simulink model "gtm_aeromodel"  (Simulink 7.2)
settings: Solver=ode45  StartTime=0.0  StopTime=10.0  RelTol=1e-3
undefined symbols (not defined in the file or in its folder): A_BLCG, A_BW, A_CW, A_FSCG, A_FSREF_in, A_SW, A_WLCG, A_WLREF, ALPHA0, bclowb, bclowbx_FMACH, bcmowb, bcmowbx_FHP, bcmowby_FMACH, cda, cdax_FLPDEF, cddr, cddrx_FMACH, cdo, cdox_FLPDEF, cdt1, cdt1x_mach, cdt2, cdt2x_mach, cdto, cdtox_mach, cdwb, cdwbx_FALPHA, cdwby_FMACH, clat, clatfr, clatfrx_FHP, clatfry_FMACH, clatx_mach, clawbfr, clawbfrx_FHP, clawbfry_FMACH, cldefr, cldefrx_FHP, cldefry_FMACH, cldtab, cldtabx_FMACH, clqwb, clqwbfr, clqwbfrx_FHP, clqwbfry_FMACH, clqwbx_mach, cltdd, cltddx_FHP, cltddy_FMACH, clwb, clwbtdd, clwbtddx_FHP, clwbtddy_FMACH, clwbx_FALPHA, clwby_FMACH, clwbzdd, clwbzddx_FHP, clwbzddy_FMACH, clzdd ... (+196)
libraries: model_lib x1
(part 5 of 10)

== system gtm_aeromodel/get aero forces and moments/AERODYNAMICS/Force  Coefficients/SIDE/CYSPOIL ==
  dsb : Inport  OutDataType=sfix(16)  OutScaling=2^0
  dsl : Inport  Port=2  OutDataType=sfix(16)  OutScaling=2^0
  alpha : Inport  Port=3  OutDataType=sfix(16)  OutScaling=2^0
  mach : Inport  Port=4  OutDataType=sfix(16)  OutScaling=2^0
  flap : Inport  Port=5  OutDataType=sfix(16)  OutScaling=2^0
  dsr : Inport  Port=6  OutDataType=sfix(16)  OutScaling=2^0
  MACH : Constant  Value=.178  OutDataType=sfix(16)  OutScaling=2^0
  Sum1 : Sum  Inputs=-+  OutDataType=sfix(16)  OutScaling=2^0  SaturateOnIntegerOverflow=on  InputSameDT=on  OutDataTypeStr=Inherit: Same as first input
  Sum2 : Sum  OutDataType=sfix(16)  OutScaling=2^0  SaturateOnIntegerOverflow=on  InputSameDT=on  OutDataTypeStr=Inherit: Same as first input
  Sum5 : Sum  Inputs=+-  OutDataType=sfix(16)  OutScaling=2^0  SaturateOnIntegerOverflow=on  InputSameDT=on  OutDataTypeStr=Inherit: Same as first input
  Sum6 : Sum  Inputs=+-  OutDataType=sfix(16)  OutScaling=2^0  SaturateOnIntegerOverflow=on  InputSameDT=on  OutDataTypeStr=Inherit: Same as first input
  Sum7 : Sum  Inputs=+-  OutDataType=sfix(16)  OutScaling=2^0  SaturateOnIntegerOverflow=on  InputSameDT=on  OutDataTypeStr=Inherit: Same as first input
  Switch7 : Switch  Threshold=0.5  SaturateOnIntegerOverflow=on  InputSameDT=on
  cy_sp_int : Subsystem  TreatAsAtomicUnit=on
  dclpfint1 : Sum  Inputs=-+  OutDataType=sfix(16)  OutScaling=2^0  SaturateOnIntegerOverflow=on  InputSameDT=on  OutDataTypeStr=Inherit: Same as first input
  dclpfint2 : Sum  Inputs=-+  OutDataType=sfix(16)  OutScaling=2^0  SaturateOnIntegerOverflow=on  InputSameDT=on  OutDataTypeStr=Inherit: Same as first input
  dcyspfint : Sum  Inputs=-+  OutDataType=sfix(16)  OutScaling=2^0  SaturateOnIntegerOverflow=on  InputSameDT=on  OutDataTypeStr=Inherit: Same as first input
  dcywbdsl : Subsystem  mask(1-2-3 Table){@1=dcywbdsl_Fx_DSL, @2=dcywbdsl_Fy_FALPHA, @3=dcywbdsl_Fz_FMACH, @4=dcywbdsl_F}
      mask prompts: @1 "X vector:"; @2 "Y vector:"; @3 "Z vector:"; @4 "Table:"
      mask help: 3-D Table Look Up. Enter monotonic X, Y and Z vectors and a matrix of 2-D tables. See the help for more info.
      mask init:
      | x=@1;y=@2;z=@3;tab=@4;
      mask Help: The X, Y and Z vectors must be monotonic.   The 3-D table is a horizontal concatenation of  2-D tables.  X  indexes into the columns of the 2-D tables & Y indexes into the rows of the 2-D tables.  Z indexes into the table levels (starting with the 1st 2-D table).   The input values are x, y and z respectively (e.g., top port = x).
      mask Display: plot([0 2 2 0 0],[0 0 2 2 0],[0 2 2.9 0.95 0],[2 2 2.7 2.7 2],[2 2.9 2.9 2 2],[0 0.85 2.7 2 0])
  dcywbdsl1 : Subsystem  mask(1-2-3 Table){@1=dcywbdsl_Fx_DSL, @2=dcywbdsl_Fy_FALPHA, @3=dcywbdsl_Fz_FMACH, @4=dcywbdsl_F}
      mask prompts: @1 "X vector:"; @2 "Y vector:"; @3 "Z vector:"; @4 "Table:"
      mask help: 3-D Table Look Up. Enter monotonic X, Y and Z vectors and a matrix of 2-D tables. See the help for more info.
      mask init:
      | x=@1;y=@2;z=@3;tab=@4;
      mask Help: The X, Y and Z vectors must be monotonic.   The 3-D table is a horizontal concatenation of  2-D tables.  X  indexes into the columns of the 2-D tables & Y indexes into the rows of the 2-D tables.  Z indexes into the table levels (starting with the 1st 2-D table).   The input values are x, y and z respectively (e.g., top port = x).
      mask Display: plot([0 2 2 0 0],[0 0 2 2 0],[0 2 2.9 0.95 0],[2 2 2.7 2.7 2],[2 2.9 2.9 2 2],[0 0.85 2.7 2 0])
  dcywbdsl2 : Subsystem  mask(1-2-3 Table){@1=dcywbdsl_Fx_DSL, @2=dcywbdsl_Fy_FALPHA, @3=dcywbdsl_Fz_FMACH, @4=dcywbdsl_F}
      mask prompts: @1 "X vector:"; @2 "Y vector:"; @3 "Z vector:"; @4 "Table:"
      mask help: 3-D Table Look Up. Enter monotonic X, Y and Z vectors and a matrix of 2-D tables. See the help for more info.
      mask init:
      | x=@1;y=@2;z=@3;tab=@4;
      mask Help: The X, Y and Z vectors must be monotonic.   The 3-D table is a horizontal concatenation of  2-D tables.  X  indexes into the columns of the 2-D tables & Y indexes into the rows of the 2-D tables.  Z indexes into the table levels (starting with the 1st 2-D table).   The input values are x, y and z respectively (e.g., top port = x).
      mask Display: plot([0 2 2 0 0],[0 0 2 2 0],[0 2 2.9 0.95 0],[2 2 2.7 2.7 2],[2 2.9 2.9 2 2],[0 0.85 2.7 2 0])
  dcywbdsl3 : Subsystem  mask(1-2-3 Table){@1=dcywbdsl_Fx_DSL, @2=dcywbdsl_Fy_FALPHA, @3=dcywbdsl_Fz_FMACH, @4=dcywbdsl_F}
      mask prompts: @1 "X vector:"; @2 "Y vector:"; @3 "Z vector:"; @4 "Table:"
      mask help: 3-D Table Look Up. Enter monotonic X, Y and Z vectors and a matrix of 2-D tables. See the help for more info.
      mask init:
      | x=@1;y=@2;z=@3;tab=@4;
      mask Help: The X, Y and Z vectors must be monotonic.   The 3-D table is a horizontal concatenation of  2-D tables.  X  indexes into the columns of the 2-D tables & Y indexes into the rows of the 2-D tables.  Z indexes into the table levels (starting with the 1st 2-D table).   The input values are x, y and z respectively (e.g., top port = x).
      mask Display: plot([0 2 2 0 0],[0 0 2 2 0],[0 2 2.9 0.95 0],[2 2 2.7 2.7 2],[2 2.9 2.9 2 2],[0 0.85 2.7 2 0])
  dcywbdsl4 : Subsystem  mask(1-2-3 Table){@1=dcywbdsl_Fx_DSL, @2=dcywbdsl_Fy_FALPHA, @3=dcywbdsl_Fz_FMACH, @4=dcywbdsl_F}
      mask prompts: @1 "X vector:"; @2 "Y vector:"; @3 "Z vector:"; @4 "Table:"
      mask help: 3-D Table Look Up. Enter monotonic X, Y and Z vectors and a matrix of 2-D tables. See the help for more info.
      mask init:
      | x=@1;y=@2;z=@3;tab=@4;
      mask Help: The X, Y and Z vectors must be monotonic.   The 3-D table is a horizontal concatenation of  2-D tables.  X  indexes into the columns of the 2-D tables & Y indexes into the rows of the 2-D tables.  Z indexes into the table levels (starting with the 1st 2-D table).   The input values are x, y and z respectively (e.g., top port = x).
      mask Display: plot([0 2 2 0 0],[0 0 2 2 0],[0 2 2.9 0.95 0],[2 2 2.7 2.7 2],[2 2.9 2.9 2 2],[0 0.85 2.7 2 0])
  dcywbdsl5 : Subsystem  mask(1-2-3 Table){@1=dcywbdsl_Fx_DSL, @2=dcywbdsl_Fy_FALPHA, @3=dcywbdsl_Fz_FMACH, @4=dcywbdsl_F}
      mask prompts: @1 "X vector:"; @2 "Y vector:"; @3 "Z vector:"; @4 "Table:"
      mask help: 3-D Table Look Up. Enter monotonic X, Y and Z vectors and a matrix of 2-D tables. See the help for more info.
      mask init:
      | x=@1;y=@2;z=@3;tab=@4;
      mask Help: The X, Y and Z vectors must be monotonic.   The 3-D table is a horizontal concatenation of  2-D tables.  X  indexes into the columns of the 2-D tables & Y indexes into the rows of the 2-D tables.  Z indexes into the table levels (starting with the 1st 2-D table).   The input values are x, y and z respectively (e.g., top port = x).
      mask Display: plot([0 2 2 0 0],[0 0 2 2 0],[0 2 2.9 0.95 0],[2 2 2.7 2.7 2],[2 2.9 2.9 2 2],[0 0.85 2.7 2 0])
  zero : Constant  Value=0.0  OutDataType=sfix(16)  OutScaling=2^0
  cy_spoil : Outport  OutDataType=sfix(16)  OutScaling=2^0  InitialOutput=0
  wires:
  Sum6/1 -> Sum2/1
  dsb/1 -> dcywbdsl1/1(X), cy_sp_int/4(dsb), dcywbdsl3/1(X)
  zero/1 -> Switch7/3
  dcywbdsl2/1(Interp Value) -> Sum5/1
  Sum1/1 -> Sum6/1
  Sum5/1 -> Sum6/2
  dsl/1 -> dcywbdsl/1(X), cy_sp_int/3(dsl), dcywbdsl4/1(X)
  alpha/1 -> dcywbdsl/2(Y), dcywbdsl2/2(Y), dcywbdsl3/2(Y), cy_sp_int/2(alpha), dcywbdsl5/2(Y), dcywbdsl4/2(Y), dcywbdsl1/2(Y)
  dcywbdsl/1(Interp Value) -> Sum1/2
  mach/1 -> dcywbdsl/3(Z), dcywbdsl1/3(Z), dcywbdsl2/3(Z)
  dsr/1 -> dcywbdsl2/1(X), dcywbdsl5/1(X), cy_sp_int/5(dsr)
  dcywbdsl5/1(Interp Value) -> dclpfint1/2
  dcywbdsl3/1(Interp Value) -> dclpfint1/1, dclpfint2/1
  dcywbdsl4/1(Interp Value) -> dclpfint2/2
  dclpfint2/1 -> Sum7/1
  dclpfint1/1 -> Sum7/2
  Sum7/1 -> dcyspfint/1
  MACH/1 -> dcywbdsl5/3(Z), dcywbdsl4/3(Z), dcywbdsl3/3(Z)
  dcywbdsl1/1(Interp Value) -> Sum1/1, Sum5/2
  flap/1 -> cy_sp_int/Enable, Switch7/2, cy_sp_int/1(flap)
  cy_sp_int/1(cy_spfl_int) -> dcyspfint/2
  dcyspfint/1 -> Switch7/1
  Sum2/1 -> cy_spoil/1
  Switch7/1 -> Sum2/2

== system gtm_aeromodel/get aero forces and moments/AERODYNAMICS/Force  Coefficients/SIDE/TAIL ==
  mach : Inport  OutDataType=sfix(16)  OutScaling=2^0
  alpha : Inport  Port=2  OutDataType=sfix(16)  OutScaling=2^0
  Sum : Sum  OutDataType=sfix(16)  OutScaling=2^0  SaturateOnIntegerOverflow=on  InputSameDT=on  OutDataTypeStr=Inherit: Same as first input
  cybht : Subsystem  mask(2-D Table){y=cybhtx_FMACH, z=cybhty_FALPHA, tab=cybht}
      mask prompts: y "Y vector:"; z "Z vector:"; tab "Table:"
      mask help: 2-D Table Look Up. Enter monotonic Y and Z vectors and a matrix of 2-D tables. See the help for more info.
      mask Help: The Y and Z vectors must be monotonic.  Y  indexes into the columns of the 2-D table & Z indexes into the rows of the 2-D tables.   The input values are y and z respectively (e.g., top port = y).
      mask Display: plot(-10,-10,110,110,[90,50,10],[90,40,30],[90,50,10],[50,26,20],[90,50,10],[22,13,10])
  cybvt : Subsystem  mask(2-D Table){y=cybvtx_FMACH, z=cybvty_FALPHA, tab=cybvt}
      mask prompts: y "Y vector:"; z "Z vector:"; tab "Table:"
      mask help: 2-D Table Look Up. Enter monotonic Y and Z vectors and a matrix of 2-D tables. See the help for more info.
      mask Help: The Y and Z vectors must be monotonic.  Y  indexes into the columns of the 2-D table & Z indexes into the rows of the 2-D tables.   The input values are y and z respectively (e.g., top port = y).
      mask Display: plot(-10,-10,110,110,[90,50,10],[90,40,30],[90,50,10],[50,26,20],[90,50,10],[22,13,10])
  cyb_ht_vt : Outport  OutDataType=sfix(16)  OutScaling=2^0  InitialOutput=0
  wires:
  alpha/1 -> cybvt/2(Z), cybht/2(Z)
  mach/1 -> cybvt/1(Y), cybht/1(Y)
  cybht/1(Interp Value) -> Sum/1
  Sum/1 -> cyb_ht_vt/1
  cybvt/1(Interp Value) -> Sum/2

== system gtm_aeromodel/get aero forces and moments/AERODYNAMICS/Moment Coefficients/PITCH/BCMOWB ==
  mach : Inport  OutDataType=sfix(16)  OutScaling=2^0
  altitude : Inport  Port=2  OutDataType=sfix(16)  OutScaling=2^0
  cmatfr : Subsystem  mask(2-D Table){y=bcmowbx_FHP, z=bcmowby_FMACH, tab=bcmowb}
      mask prompts: y "Y vector:"; z "Z vector:"; tab "Table:"
      mask help: 2-D Table Look Up. Enter monotonic Y and Z vectors and a matrix of 2-D tables. See the help for more info.
      mask Help: The Y and Z vectors must be monotonic.  Y  indexes into the columns of the 2-D table & Z indexes into the rows of the 2-D tables.   The input values are y and z respectively (e.g., top port = y).
      mask Display: plot(-10,-10,110,110,[90,50,10],[90,40,30],[90,50,10],[50,26,20],[90,50,10],[22,13,10])
  bcmowb : Outport  OutDataType=sfix(16)  OutScaling=2^0  InitialOutput=0
  wires:
  cmatfr/1(Interp Value) -> bcmowb/1
  mach/1 -> cmatfr/2(Z)
  altitude/1 -> cmatfr/1(Y)

== system gtm_aeromodel/get aero forces and moments/AERODYNAMICS/Moment Coefficients/PITCH/CMQWB ==
  mach : Inport  OutDataType=sfix(16)  OutScaling=2^0
  qhat : Inport  Port=2  OutDataType=sfix(16)  OutScaling=2^0
  flex : Inport  Port=3  OutDataType=sfix(16)  OutScaling=2^0
  altitude : Inport  Port=4  OutDataType=sfix(16)  OutScaling=2^0
  Product : Product  Inputs=3  OutDataType=sfix(16)  OutScaling=2^0  SaturateOnIntegerOverflow=on  RndMeth=Zero  InputSameDT=on  OutDataTypeStr=Inherit: Same as first input
  Switch5 : Switch  Threshold=0.5  SaturateOnIntegerOverflow=on  InputSameDT=on
  cmqwb_ : Subsystem  mask(1-D Table){z=cmqwbx_mach, tab=cmqwb}
      mask prompts: z "Z vector:"; tab "Table:"
      mask help: 1-D Table Look Up. Enter monotonic Z vector amd table. See the help for more info.
      mask Help: The Z vector must be monotonic.  Z indexes into the columns of the 1-D tables.   Table does not extrapolate beyound the break vectors
      mask Display: plot(@2)
  cmqwbfr : Subsystem  TreatAsAtomicUnit=on
  one : Constant  Value=1.0  OutDataType=sfix(16)  OutScaling=2^0
  dcmqwb : Outport  OutDataType=sfix(16)  OutScaling=2^0  InitialOutput=0
  wires:
  mach/1 -> cmqwbfr/2(mach1), cmqwb_/1(Z)
  altitude/1 -> cmqwbfr/1(altitude)
  Switch5/1 -> Product/3
  one/1 -> Switch5/3
  flex/1 -> Switch5/2, cmqwbfr/Enable
  cmqwbfr/1(cmqwbfr) -> Switch5/1
  cmqwb_/1(Interp Value) -> Product/1
  qhat/1 -> Product/2
  Product/1 -> dcmqwb/1

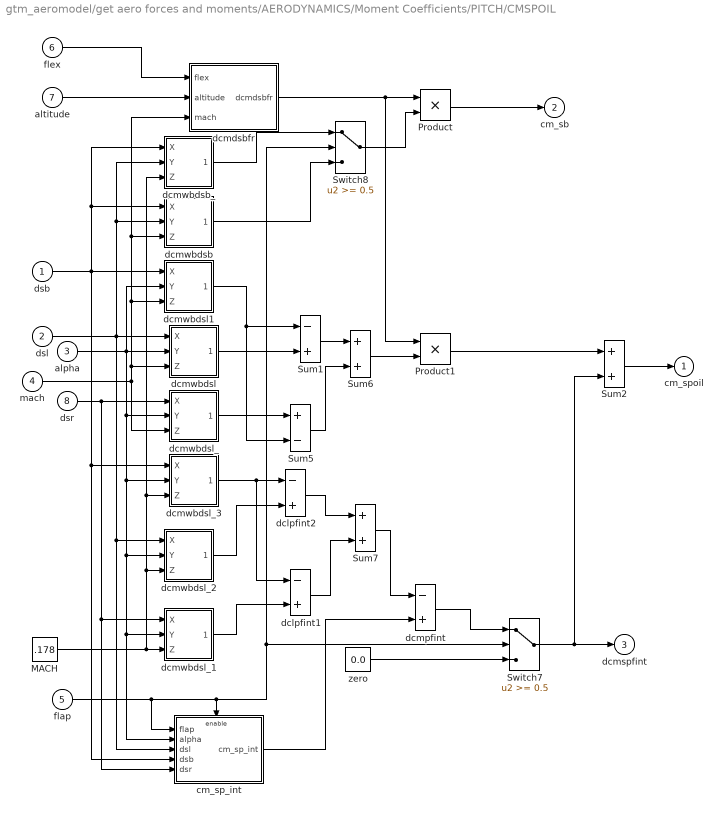
== system gtm_aeromodel/get aero forces and moments/AERODYNAMICS/Moment Coefficients/PITCH/CMSPOIL ==
  dsb : Inport  OutDataType=sfix(16)  OutScaling=2^0
  dsl : Inport  Port=2  OutDataType=sfix(16)  OutScaling=2^0
  alpha : Inport  Port=3  OutDataType=sfix(16)  OutScaling=2^0
  mach : Inport  Port=4  OutDataType=sfix(16)  OutScaling=2^0
  flap : Inport  Port=5  OutDataType=sfix(16)  OutScaling=2^0
  flex : Inport  Port=6  OutDataType=sfix(16)  OutScaling=2^0
  altitude : Inport  Port=7  OutDataType=sfix(16)  OutScaling=2^0
  dsr : Inport  Port=8  OutDataType=sfix(16)  OutScaling=2^0
  MACH : Constant  Value=.178  OutDataType=sfix(16)  OutScaling=2^0
  Product : Product  OutDataType=sfix(16)  OutScaling=2^0  SaturateOnIntegerOverflow=on  RndMeth=Zero  InputSameDT=on  OutDataTypeStr=Inherit: Same as first input
  Product1 : Product  OutDataType=sfix(16)  OutScaling=2^0  SaturateOnIntegerOverflow=on  RndMeth=Zero  InputSameDT=on  OutDataTypeStr=Inherit: Same as first input
  Sum1 : Sum  Inputs=-+  OutDataType=sfix(16)  OutScaling=2^0  SaturateOnIntegerOverflow=on  InputSameDT=on  OutDataTypeStr=Inherit: Same as first input
  Sum2 : Sum  OutDataType=sfix(16)  OutScaling=2^0  SaturateOnIntegerOverflow=on  InputSameDT=on  OutDataTypeStr=Inherit: Same as first input
  Sum5 : Sum  Inputs=+-  OutDataType=sfix(16)  OutScaling=2^0  SaturateOnIntegerOverflow=on  InputSameDT=on  OutDataTypeStr=Inherit: Same as first input
  Sum6 : Sum  OutDataType=sfix(16)  OutScaling=2^0  SaturateOnIntegerOverflow=on  InputSameDT=on  OutDataTypeStr=Inherit: Same as first input
  Sum7 : Sum  OutDataType=sfix(16)  OutScaling=2^0  SaturateOnIntegerOverflow=on  InputSameDT=on  OutDataTypeStr=Inherit: Same as first input
  Switch7 : Switch  Threshold=0.5  SaturateOnIntegerOverflow=on  InputSameDT=on
  Switch8 : Switch  Threshold=0.5  SaturateOnIntegerOverflow=on  InputSameDT=on
  cm_sp_int : Subsystem  TreatAsAtomicUnit=on
  dclpfint1 : Sum  Inputs=-+  OutDataType=sfix(16)  OutScaling=2^0  SaturateOnIntegerOverflow=on  InputSameDT=on  OutDataTypeStr=Inherit: Same as first input
  dclpfint2 : Sum  Inputs=-+  OutDataType=sfix(16)  OutScaling=2^0  SaturateOnIntegerOverflow=on  InputSameDT=on  OutDataTypeStr=Inherit: Same as first input
  dcmdsbfr : Subsystem
  dcmpfint : Sum  Inputs=-+  OutDataType=sfix(16)  OutScaling=2^0  SaturateOnIntegerOverflow=on  InputSameDT=on  OutDataTypeStr=Inherit: Same as first input
  dcmwbdsb : Subsystem  mask(1-2-3 Table){@1=dcmwbdsbx_DSB, @2=dcmwbdsby_ALPHA, @3=dcmwbdsbz_FMACH, @4=dcmwbdsb}
      mask prompts: @1 "X vector:"; @2 "Y vector:"; @3 "Z vector:"; @4 "Table:"
      mask help: 3-D Table Look Up. Enter monotonic X, Y and Z vectors and a matrix of 2-D tables. See the help for more info.
      mask init:
      | x=@1;y=@2;z=@3;tab=@4;
      mask Help: The X, Y and Z vectors must be monotonic.   The 3-D table is a horizontal concatenation of  2-D tables.  X  indexes into the columns of the 2-D tables & Y indexes into the rows of the 2-D tables.  Z indexes into the table levels (starting with the 1st 2-D table).   The input values are x, y and z respectively (e.g., top port = x).
      mask Display: plot([0 2 2 0 0],[0 0 2 2 0],[0 2 2.9 0.95 0],[2 2 2.7 2.7 2],[2 2.9 2.9 2 2],[0 0.85 2.7 2 0])
  dcmwbdsb_ : Subsystem  mask(1-2-3 Table){@1=dcmwbdsbx_DSB, @2=dcmwbdsby_ALPHA, @3=dcmwbdsbz_FMACH, @4=dcmwbdsb}
      mask prompts: @1 "X vector:"; @2 "Y vector:"; @3 "Z vector:"; @4 "Table:"
      mask help: 3-D Table Look Up. Enter monotonic X, Y and Z vectors and a matrix of 2-D tables. See the help for more info.
      mask init:
      | x=@1;y=@2;z=@3;tab=@4;
      mask Help: The X, Y and Z vectors must be monotonic.   The 3-D table is a horizontal concatenation of  2-D tables.  X  indexes into the columns of the 2-D tables & Y indexes into the rows of the 2-D tables.  Z indexes into the table levels (starting with the 1st 2-D table).   The input values are x, y and z respectively (e.g., top port = x).
      mask Display: plot([0 2 2 0 0],[0 0 2 2 0],[0 2 2.9 0.95 0],[2 2 2.7 2.7 2],[2 2.9 2.9 2 2],[0 0.85 2.7 2 0])
  dcmwbdsl : Subsystem  mask(1-2-3 Table){@1=dcmwbdslx_DSL, @2=dcmwbdsly_FALPHA, @3=dcmwbdslz_FMACH, @4=dcmwbdsl}
      mask prompts: @1 "X vector:"; @2 "Y vector:"; @3 "Z vector:"; @4 "Table:"
      mask help: 3-D Table Look Up. Enter monotonic X, Y and Z vectors and a matrix of 2-D tables. See the help for more info.
      mask init:
      | x=@1;y=@2;z=@3;tab=@4;
      mask Help: The X, Y and Z vectors must be monotonic.   The 3-D table is a horizontal concatenation of  2-D tables.  X  indexes into the columns of the 2-D tables & Y indexes into the rows of the 2-D tables.  Z indexes into the table levels (starting with the 1st 2-D table).   The input values are x, y and z respectively (e.g., top port = x).
      mask Display: plot([0 2 2 0 0],[0 0 2 2 0],[0 2 2.9 0.95 0],[2 2 2.7 2.7 2],[2 2.9 2.9 2 2],[0 0.85 2.7 2 0])
  dcmwbdsl1 : Subsystem  mask(1-2-3 Table){@1=dcmwbdslx_DSL, @2=dcmwbdsly_FALPHA, @3=dcmwbdslz_FMACH, @4=dcmwbdsl}
      mask prompts: @1 "X vector:"; @2 "Y vector:"; @3 "Z vector:"; @4 "Table:"
      mask help: 3-D Table Look Up. Enter monotonic X, Y and Z vectors and a matrix of 2-D tables. See the help for more info.
      mask init:
      | x=@1;y=@2;z=@3;tab=@4;
      mask Help: The X, Y and Z vectors must be monotonic.   The 3-D table is a horizontal concatenation of  2-D tables.  X  indexes into the columns of the 2-D tables & Y indexes into the rows of the 2-D tables.  Z indexes into the table levels (starting with the 1st 2-D table).   The input values are x, y and z respectively (e.g., top port = x).
      mask Display: plot([0 2 2 0 0],[0 0 2 2 0],[0 2 2.9 0.95 0],[2 2 2.7 2.7 2],[2 2.9 2.9 2 2],[0 0.85 2.7 2 0])
  dcmwbdsl_ : Subsystem  mask(1-2-3 Table){@1=dcmwbdslx_DSL, @2=dcmwbdsly_FALPHA, @3=dcmwbdslz_FMACH, @4=dcmwbdsl}
      mask prompts: @1 "X vector:"; @2 "Y vector:"; @3 "Z vector:"; @4 "Table:"
      mask help: 3-D Table Look Up. Enter monotonic X, Y and Z vectors and a matrix of 2-D tables. See the help for more info.
      mask init:
      | x=@1;y=@2;z=@3;tab=@4;
      mask Help: The X, Y and Z vectors must be monotonic.   The 3-D table is a horizontal concatenation of  2-D tables.  X  indexes into the columns of the 2-D tables & Y indexes into the rows of the 2-D tables.  Z indexes into the table levels (starting with the 1st 2-D table).   The input values are x, y and z respectively (e.g., top port = x).
      mask Display: plot([0 2 2 0 0],[0 0 2 2 0],[0 2 2.9 0.95 0],[2 2 2.7 2.7 2],[2 2.9 2.9 2 2],[0 0.85 2.7 2 0])
  dcmwbdsl_1 : Subsystem  mask(1-2-3 Table){@1=dcmwbdslx_DSL, @2=dcmwbdsly_FALPHA, @3=dcmwbdslz_FMACH, @4=dcmwbdsl}
      mask prompts: @1 "X vector:"; @2 "Y vector:"; @3 "Z vector:"; @4 "Table:"
      mask help: 3-D Table Look Up. Enter monotonic X, Y and Z vectors and a matrix of 2-D tables. See the help for more info.
      mask init:
      | x=@1;y=@2;z=@3;tab=@4;
      mask Help: The X, Y and Z vectors must be monotonic.   The 3-D table is a horizontal concatenation of  2-D tables.  X  indexes into the columns of the 2-D tables & Y indexes into the rows of the 2-D tables.  Z indexes into the table levels (starting with the 1st 2-D table).   The input values are x, y and z respectively (e.g., top port = x).
      mask Display: plot([0 2 2 0 0],[0 0 2 2 0],[0 2 2.9 0.95 0],[2 2 2.7 2.7 2],[2 2.9 2.9 2 2],[0 0.85 2.7 2 0])
  dcmwbdsl_2 : Subsystem  mask(1-2-3 Table){@1=dcmwbdslx_DSL, @2=dcmwbdsly_FALPHA, @3=dcmwbdslz_FMACH, @4=dcmwbdsl}
      mask prompts: @1 "X vector:"; @2 "Y vector:"; @3 "Z vector:"; @4 "Table:"
      mask help: 3-D Table Look Up. Enter monotonic X, Y and Z vectors and a matrix of 2-D tables. See the help for more info.
      mask init:
      | x=@1;y=@2;z=@3;tab=@4;
      mask Help: The X, Y and Z vectors must be monotonic.   The 3-D table is a horizontal concatenation of  2-D tables.  X  indexes into the columns of the 2-D tables & Y indexes into the rows of the 2-D tables.  Z indexes into the table levels (starting with the 1st 2-D table).   The input values are x, y and z respectively (e.g., top port = x).
      mask Display: plot([0 2 2 0 0],[0 0 2 2 0],[0 2 2.9 0.95 0],[2 2 2.7 2.7 2],[2 2.9 2.9 2 2],[0 0.85 2.7 2 0])
  dcmwbdsl_3 : Subsystem  mask(1-2-3 Table){@1=dcmwbdslx_DSL, @2=dcmwbdsly_FALPHA, @3=dcmwbdslz_FMACH, @4=dcmwbdsl}
      mask prompts: @1 "X vector:"; @2 "Y vector:"; @3 "Z vector:"; @4 "Table:"
      mask help: 3-D Table Look Up. Enter monotonic X, Y and Z vectors and a matrix of 2-D tables. See the help for more info.
      mask init:
      | x=@1;y=@2;z=@3;tab=@4;
      mask Help: The X, Y and Z vectors must be monotonic.   The 3-D table is a horizontal concatenation of  2-D tables.  X  indexes into the columns of the 2-D tables & Y indexes into the rows of the 2-D tables.  Z indexes into the table levels (starting with the 1st 2-D table).   The input values are x, y and z respectively (e.g., top port = x).
      mask Display: plot([0 2 2 0 0],[0 0 2 2 0],[0 2 2.9 0.95 0],[2 2 2.7 2.7 2],[2 2.9 2.9 2 2],[0 0.85 2.7 2 0])
  zero : Constant  Value=0.0  OutDataType=sfix(16)  OutScaling=2^0
  cm_spoil : Outport  OutDataType=sfix(16)  OutScaling=2^0  InitialOutput=0
  cm_sb : Outport  Port=2  OutDataType=sfix(16)  OutScaling=2^0  InitialOutput=0
  dcmspfint : Outport  Port=3  OutDataType=sfix(16)  OutScaling=2^0  InitialOutput=0
  wires:
  flex/1 -> dcmdsbfr/1(flex)
  dcmwbdsb_/1(Interp Value) -> Switch8/1
  dcmwbdsb/1(Interp Value) -> Switch8/3
  dcmwbdsl1/1(Interp Value) -> Sum5/2, Sum1/1
  MACH/1 -> dcmwbdsb_/3(Z), dcmwbdsl_3/3(Z), dcmwbdsl_2/3(Z), dcmwbdsl_1/3(Z)
  Sum7/1 -> dcmpfint/1
  dclpfint1/1 -> Sum7/2
  dclpfint2/1 -> Sum7/1
  dcmwbdsl_2/1(Interp Value) -> dclpfint2/2
  dcmwbdsl_3/1(Interp Value) -> dclpfint2/1, dclpfint1/1
  dcmwbdsl_1/1(Interp Value) -> dclpfint1/2
  dsr/1 -> cm_sp_int/5(dsr), dcmwbdsl_1/1(X), dcmwbdsl_/1(X)
  mach/1 -> dcmwbdsl_/3(Z), dcmwbdsb/3(Z), dcmdsbfr/3(mach), dcmwbdsl1/3(Z), dcmwbdsl/3(Z)
  dcmwbdsl/1(Interp Value) -> Sum1/2
  alpha/1 -> dcmwbdsl1/2(Y), dcmwbdsl_2/2(Y), dcmwbdsl_1/2(Y), cm_sp_int/2(alpha), dcmwbdsl_3/2(Y), dcmwbdsl_/2(Y), dcmwbdsl/2(Y)
  dsl/1 -> dcmwbdsb_/2(Y), dcmwbdsb/2(Y), dcmwbdsl_2/1(X), cm_sp_int/3(dsl), dcmwbdsl/1(X)
  Sum6/1 -> Product1/2
  Sum5/1 -> Sum6/2
  Sum1/1 -> Sum6/1
  dcmwbdsl_/1(Interp Value) -> Sum5/1
  Product1/1 -> Sum2/1
  Sum2/1 -> cm_spoil/1
  flap/1 -> cm_sp_int/1(flap), Switch8/2, Switch7/2, cm_sp_int/Enable
  zero/1 -> Switch7/3
  dsb/1 -> dcmwbdsb_/1(X), dcmwbdsb/1(X), dcmwbdsl_3/1(X), cm_sp_int/4(dsb), dcmwbdsl1/1(X)
  dcmdsbfr/1(dcmdsbfr) -> Product1/1, Product/1
  Product/1 -> cm_sb/1
  Switch8/1 -> Product/2
  altitude/1 -> dcmdsbfr/2(altitude)
  cm_sp_int/1(cm_sp_int) -> dcmpfint/2
  dcmpfint/1 -> Switch7/1
  Switch7/1 -> Sum2/2, dcmspfint/1

== system gtm_aeromodel/get aero forces and moments/AERODYNAMICS/Moment Coefficients/PITCH/CMT ==
  mach : Inport  OutDataType=sfix(16)  OutScaling=2^0
  alphat : Inport  Port=2  OutDataType=sfix(16)  OutScaling=2^0
  altitude : Inport  Port=3  OutDataType=sfix(16)  OutScaling=2^0
  norm acc g's : Inport  Port=4  OutDataType=sfix(16)  OutScaling=2^0
  qdot : Inport  Port=5  OutDataType=sfix(16)  OutScaling=2^0
  flex : Inport  Port=6  OutDataType=sfix(16)  OutScaling=2^0
  CMAT : Subsystem  mask(1-D Table){z=CMATx_mach, tab=CMAT}
      mask prompts: z "Z vector:"; tab "Table:"
      mask help: 1-D Table Look Up. Enter monotonic Z vector amd table. See the help for more info.
      mask Help: The Z vector must be monotonic.  Z indexes into the columns of the 1-D tables.   Table does not extrapolate beyound the break vectors
      mask Display: plot(@2)
  Product : Product  OutDataType=sfix(16)  OutScaling=2^0  SaturateOnIntegerOverflow=on  RndMeth=Zero  InputSameDT=on  OutDataTypeStr=Inherit: Same as first input
  Product1 : Product  OutDataType=sfix(16)  OutScaling=2^0  SaturateOnIntegerOverflow=on  RndMeth=Zero  InputSameDT=on  OutDataTypeStr=Inherit: Same as first input
  R2D3 : Gain  ParameterDataType=sfix(16)  ParameterScaling=2^0  OutDataType=sfix(16)  OutScaling=2^0  SaturateOnIntegerOverflow=on  OutDataTypeStr=Inherit: Same as input  ParamDataTypeStr=Inherit: Same as input
  Sum : Sum  OutDataType=sfix(16)  OutScaling=2^0  SaturateOnIntegerOverflow=on  InputSameDT=on  OutDataTypeStr=Inherit: Same as first input
  Switch6 : Switch  Threshold=0.5  SaturateOnIntegerOverflow=on  InputSameDT=on
  Switch7 : Switch  Threshold=0.5  SaturateOnIntegerOverflow=on  InputSameDT=on
  cltailfx : Subsystem  TreatAsAtomicUnit=on
  constant1 : Constant  Value=0.0  OutDataType=sfix(16)  OutScaling=2^0
  constant2 : Constant  OutDataType=sfix(16)  OutScaling=2^0
  cmt : Outport  OutDataType=sfix(16)  OutScaling=2^0
  wires:
  Switch7/1 -> Product1/2
  Switch6/1 -> Sum/2
  Product/1 -> Sum/1
  Product1/1 -> Product/1
  CMAT/1(Interp Value) -> Product1/1
  qdot/1 -> cltailfx/4(qdot)
  norm acc g's/1 -> cltailfx/3(norm acc g's)
  cltailfx/2(cmtflx) -> Switch6/1
  flex/1 -> Switch6/2, cltailfx/Enable, Switch7/2
  constant1/1 -> Switch6/3
  mach/1 -> cltailfx/2(Mach), CMAT/1(Z)
  altitude/1 -> cltailfx/1(altitude)
  cltailfx/1(cmatfr) -> Switch7/1
  constant2/1 -> Switch7/3
  R2D3/1 -> Product/2
  alphat/1 -> R2D3/1
  Sum/1 -> cmt/1

== system gtm_aeromodel/get aero forces and moments/AERODYNAMICS/Moment Coefficients/PITCH/CMTAB ==
  mach : Inport  OutDataType=sfix(16)  OutScaling=2^0
  eletab : Inport  Port=2  OutDataType=sfix(16)  OutScaling=2^0
  alt : Inport  Port=3  OutDataType=sfix(16)  OutScaling=2^0
  flex : Inport  Port=4  OutDataType=sfix(16)  OutScaling=2^0
  Product : Product  OutDataType=sfix(16)  OutScaling=2^0  SaturateOnIntegerOverflow=on  RndMeth=Zero  InputSameDT=on  OutDataTypeStr=Inherit: Same as first input
  Product1 : Product  OutDataType=sfix(16)  OutScaling=2^0  SaturateOnIntegerOverflow=on  RndMeth=Zero  InputSameDT=on  OutDataTypeStr=Inherit: Same as first input
  Switch5 : Switch  Threshold=0.5  SaturateOnIntegerOverflow=on  InputSameDT=on
  cmdetabfr : Subsystem  TreatAsAtomicUnit=on
  cmdtab_ : Subsystem  mask(1-D Table){z=cmdtabx_FMACH, tab=cmdtab}
      mask prompts: z "Z vector:"; tab "Table:"
      mask help: 1-D Table Look Up. Enter monotonic Z vector amd table. See the help for more info.
      mask Help: The Z vector must be monotonic.  Z indexes into the columns of the 1-D tables.   Table does not extrapolate beyound the break vectors
      mask Display: plot(@2)
  zero4 : Constant  OutDataType=sfix(16)  OutScaling=2^0
  cmtab : Outport  OutDataType=sfix(16)  OutScaling=2^0  InitialOutput=0
  wires:
  flex/1 -> Switch5/2, cmdetabfr/Enable
  mach/1 -> cmdtab_/1(Z), cmdetabfr/2(mach)
  Switch5/1 -> Product1/1
  zero4/1 -> Switch5/3
  Product/1 -> cmtab/1
  alt/1 -> cmdetabfr/1(alt)
  eletab/1 -> Product/2
  cmdetabfr/1(Out1) -> Switch5/1
  Product1/1 -> Product/1
  cmdtab_/1(Interp Value) -> Product1/2

== system gtm_aeromodel/get aero forces and moments/AERODYNAMICS/Moment Coefficients/PITCH/CMWB ==
  alpha : Inport  OutDataType=sfix(16)  OutScaling=2^0
  mach : Inport  Port=2  OutDataType=sfix(16)  OutScaling=2^0
  flap : Inport  Port=3  OutDataType=sfix(16)  OutScaling=2^0
  flex : Inport  Port=4  OutDataType=sfix(16)  OutScaling=2^0
  altitude : Inport  Port=5  OutDataType=sfix(16)  OutScaling=2^0
  qdyn : Inport  Port=6  OutDataType=sfix(16)  OutScaling=2^0
  norm acc g's : Inport  Port=7  OutDataType=sfix(16)  OutScaling=2^0
  qdot : Inport  Port=8  OutDataType=sfix(16)  OutScaling=2^0
  dsb : Inport  Port=9  OutDataType=sfix(16)  OutScaling=2^0
  CMWBFLEX : Subsystem  TreatAsAtomicUnit=on
  Product1 : Product  OutDataType=sfix(16)  OutScaling=2^0  SaturateOnIntegerOverflow=on  RndMeth=Zero  InputSameDT=on  OutDataTypeStr=Inherit: Same as first input
  Sum1 : Sum  OutDataType=sfix(16)  OutScaling=2^0  SaturateOnIntegerOverflow=on  InputSameDT=on  OutDataTypeStr=Inherit: Same as first input
  Sum2 : Sum  Inputs=+-  OutDataType=sfix(16)  OutScaling=2^0  SaturateOnIntegerOverflow=on  InputSameDT=on  OutDataTypeStr=Inherit: Same as first input
  Sum3 : Sum  OutDataType=sfix(16)  OutScaling=2^0  SaturateOnIntegerOverflow=on  InputSameDT=on  OutDataTypeStr=Inherit: Same as first input
  Switch{5..6,8,10} (4 alike) : Switch  Threshold=0.5  SaturateOnIntegerOverflow=on  InputSameDT=on
  Terminator : Terminator
  cm_flap_ : Subsystem  TreatAsAtomicUnit=on
  cmwb_ : Subsystem  mask(2-D Table){y=cmwbx_FALPHA, z=cmwby_FMACH, tab=cmwb}
      mask prompts: y "Y vector:"; z "Z vector:"; tab "Table:"
      mask help: 2-D Table Look Up. Enter monotonic Y and Z vectors and a matrix of 2-D tables. See the help for more info.
      mask Help: The Y and Z vectors must be monotonic.  Y  indexes into the columns of the 2-D table & Z indexes into the rows of the 2-D tables.   The input values are y and z respectively (e.g., top port = y).
      mask Display: plot(-10,-10,110,110,[90,50,10],[90,40,30],[90,50,10],[50,26,20],[90,50,10],[22,13,10])
  cmwb_zero : Subsystem  mask(2-D Table){y=cmwbx_FALPHA, z=cmwby_FMACH, tab=cmwb}
      mask prompts: y "Y vector:"; z "Z vector:"; tab "Table:"
      mask help: 2-D Table Look Up. Enter monotonic Y and Z vectors and a matrix of 2-D tables. See the help for more info.
      mask Help: The Y and Z vectors must be monotonic.  Y  indexes into the columns of the 2-D table & Z indexes into the rows of the 2-D tables.   The input values are y and z respectively (e.g., top port = y).
      mask Display: plot(-10,-10,110,110,[90,50,10],[90,40,30],[90,50,10],[50,26,20],[90,50,10],[22,13,10])
  constant1 : Constant  Value=0.0  OutDataType=sfix(16)  OutScaling=2^0
  constant3 : Constant  Value=1.0  OutDataType=sfix(16)  OutScaling=2^0
  zero : Constant  Value=0.0  OutDataType=sfix(16)  OutScaling=2^0
  zero_ : Constant  Value=0.0  OutDataType=sfix(16)  OutScaling=2^0
  cmwb : Outport  OutDataType=sfix(16)  OutScaling=2^0  InitialOutput=0
  cm_flap : Outport  Port=2  OutDataType=sfix(16)  OutScaling=2^0  InitialOutput=0
  dcmsbfint : Outport  Port=3  OutDataType=sfix(16)  OutScaling=2^0  InitialOutput=0
  cm_flx : Outport  Port=4  OutDataType=sfix(16)  OutScaling=2^0  InitialOutput=0
  wires:
  CMWBFLEX/2(cmawbfr) -> Switch8/1
  CMWBFLEX/1(cm_flx) -> cm_flx/1
  Sum1/1 -> Sum3/2
  Switch10/1 -> dcmsbfint/1
  cm_flap_/2(dcmsbfint) -> Switch10/1
  dsb/1 -> cm_flap_/5(dsb)
  Sum2/1 -> Product1/1
  Switch8/1 -> Product1/2
  flex/1 -> cm_flap_/4(flex), Switch8/2, Switch6/2, CMWBFLEX/Enable
  qdot/1 -> CMWBFLEX/4(qdot)
  norm acc g's/1 -> CMWBFLEX/3(NZB g's)
  cmwb_zero/1(Interp Value) -> Sum2/2, Sum1/2
  zero/1 -> cmwb_zero/1(Y)
  altitude/1 -> CMWBFLEX/1(altitude)
  constant3/1 -> Switch8/3
  Sum3/1 -> cmwb/1
  cmwb_/1(Interp Value) -> Sum2/1
  qdyn/1 -> cm_flap_/3(qdyn)
  alpha/1 -> cm_flap_/2(alpha), cmwb_/1(Y)
  mach/1 -> cmwb_zero/2(Z), CMWBFLEX/2(Mach), cmwb_/2(Z)
  cm_flap_/1(cm_flap) -> Switch5/1
  flap/1 -> cm_flap_/1(flap), cm_flap_/Enable, Switch5/2, Switch10/2
  zero_/1 -> Switch5/3, Switch10/3
  Switch5/1 -> cm_flap/1
  Product1/1 -> Sum3/1
  Switch6/1 -> Sum1/1
  constant1/1 -> Switch6/3, Switch6/1
  CMWBFLEX/3(fdcmowb) -> Terminator/1

== system gtm_aeromodel/get aero forces and moments/AERODYNAMICS/Moment Coefficients/PITCH/DCMDE ==
  elev : Inport  OutDataType=sfix(16)  OutScaling=2^0
  alphat : Inport  Port=2  OutDataType=sfix(16)  OutScaling=2^0
  mach : Inport  Port=3  OutDataType=sfix(16)  OutScaling=2^0
  flex : Inport  Port=4  OutDataType=sfix(16)  OutScaling=2^0
  altitude : Inport  Port=5  OutDataType=sfix(16)  OutScaling=2^0
  Product : Product  OutDataType=sfix(16)  OutScaling=2^0  SaturateOnIntegerOverflow=on  RndMeth=Zero  InputSameDT=on  OutDataTypeStr=Inherit: Same as first input
  Switch5 : Switch  Threshold=0.5  SaturateOnIntegerOverflow=on  InputSameDT=on
  cmdefr : Subsystem  TreatAsAtomicUnit=on
  constant3 : Constant  Value=1.0  OutDataType=sfix(16)  OutScaling=2^0
  dcmde_ : Subsystem  mask(1-2-3 Table){@1=dcmdex_FELE, @2=dcmdey_ALPHAT, @3=dcmdez_FMACH, @4=dcmde}
      mask prompts: @1 "X vector:"; @2 "Y vector:"; @3 "Z vector:"; @4 "Table:"
      mask help: 3-D Table Look Up. Enter monotonic X, Y and Z vectors and a matrix of 2-D tables. See the help for more info.
      mask init:
      | x=@1;y=@2;z=@3;tab=@4;
      mask Help: The X, Y and Z vectors must be monotonic.   The 3-D table is a horizontal concatenation of  2-D tables.  X  indexes into the columns of the 2-D tables & Y indexes into the rows of the 2-D tables.  Z indexes into the table levels (starting with the 1st 2-D table).   The input values are x, y and z respectively (e.g., top port = x).
      mask Display: plot([0 2 2 0 0],[0 0 2 2 0],[0 2 2.9 0.95 0],[2 2 2.7 2.7 2],[2 2.9 2.9 2 2],[0 0.85 2.7 2 0])
  dcmde : Outport  OutDataType=sfix(16)  OutScaling=2^0  InitialOutput=0
  wires:
  constant3/1 -> Switch5/3
  Switch5/1 -> Product/2
  Product/1 -> dcmde/1
  dcmde_/1(Interp Value) -> Product/1
  flex/1 -> Switch5/2, cmdefr/Enable
  cmdefr/1(cmdefr) -> Switch5/1
  altitude/1 -> cmdefr/1(altitude)
  mach/1 -> cmdefr/2(mach), dcmde_/3(Z)
  elev/1 -> dcmde_/1(X)
  alphat/1 -> dcmde_/2(Y)

== system gtm_aeromodel/get aero forces and moments/AERODYNAMICS/Moment Coefficients/PITCH/bcmdf ==
  flap : Inport  OutDataType=sfix(16)  OutScaling=2^0
  alpha : Inport  Port=2  OutDataType=sfix(16)  OutScaling=2^0
  Logical Operator : Logic  AllPortsSameDT=off
  Logical Operator1 : Logic
  Product : Product  OutDataType=sfix(16)  OutScaling=2^0  SaturateOnIntegerOverflow=on  RndMeth=Zero  InputSameDT=on  OutDataTypeStr=Inherit: Same as first input
  Product2 : Product  Inputs=4  OutDataType=sfix(16)  OutScaling=2^0  SaturateOnIntegerOverflow=on  RndMeth=Zero  InputSameDT=on  OutDataTypeStr=Inherit: Same as first input
  Relational Operator1 : RelationalOperator  Operator=<=  InputSameDT=on
  Relational Operator2 : RelationalOperator  Operator=>  InputSameDT=on
  Relational Operator3 : RelationalOperator  Operator=<=  InputSameDT=on
  Relational Operator4 : RelationalOperator  Operator=>  InputSameDT=on
  Sum : Sum  Inputs=+++  OutDataType=sfix(16)  OutScaling=2^0  SaturateOnIntegerOverflow=on  InputSameDT=on  OutDataTypeStr=Inherit: Same as first input
  Sum5 : Sum  Inputs=-+  OutDataType=sfix(16)  OutScaling=2^0  SaturateOnIntegerOverflow=on  InputSameDT=on  OutDataTypeStr=Inherit: Same as first input
  Switch5 : Switch  Threshold=0.5  SaturateOnIntegerOverflow=on  InputSameDT=on
  Switch6 : Switch  Threshold=0.5  SaturateOnIntegerOverflow=on  InputSameDT=on
  Switch7 : Switch  Threshold=0.5  SaturateOnIntegerOverflow=on  InputSameDT=on
  zero : Constant  Value=0  OutDataType=sfix(16)  OutScaling=2^0
  zero1 : Constant  Value=10  OutDataType=sfix(16)  OutScaling=2^0
  zero2 : Constant  Value=0  OutDataType=sfix(16)  OutScaling=2^0
  zero3 : Constant  Value=-.0020  OutDataType=sfix(16)  OutScaling=2^0
  zero4 : Constant  Value=.0045  OutDataType=sfix(16)  OutScaling=2^0
  zero5 : Constant  Value=20  OutDataType=sfix(16)  OutScaling=2^0
  zero8 : Constant  Value=20  OutDataType=sfix(16)  OutScaling=2^0
  zero9 : Constant  Value=1/19  OutDataType=sfix(16)  OutScaling=2^0
  bcmdf : Outport  OutDataType=sfix(16)  OutScaling=2^0  InitialOutput=0
  wires:
  Sum5/1 -> Product2/3
  zero9/1 -> Product2/2
  Switch7/1 -> Sum/3
  Switch6/1 -> Sum/2
  Switch5/1 -> Sum/1
  Relational Operator4/1 -> Switch7/2
  zero5/1 -> Relational Operator4/2, Relational Operator3/2
  Sum/1 -> bcmdf/1
  zero2/1 -> Switch7/3, Switch6/3, Switch6/1, Switch5/3
  Logical Operator1/1 -> Switch6/2
  Relational Operator3/1 -> Logical Operator1/2
  Relational Operator2/1 -> Logical Operator1/1
  zero1/1 -> Relational Operator2/2, Relational Operator1/2
  zero/1 -> Logical Operator/1
  Logical Operator/1 -> Switch5/2
  Relational Operator1/1 -> Logical Operator/2
  zero3/1 -> Product/1
  flap/1 -> Relational Operator4/1, Relational Operator3/1, Relational Operator2/1, Relational Operator1/1, Sum5/2
  zero8/1 -> Sum5/1
  Product/1 -> Switch5/1
  Product2/1 -> Switch7/1
  alpha/1 -> Product/2, Product2/1
  zero4/1 -> Product2/4

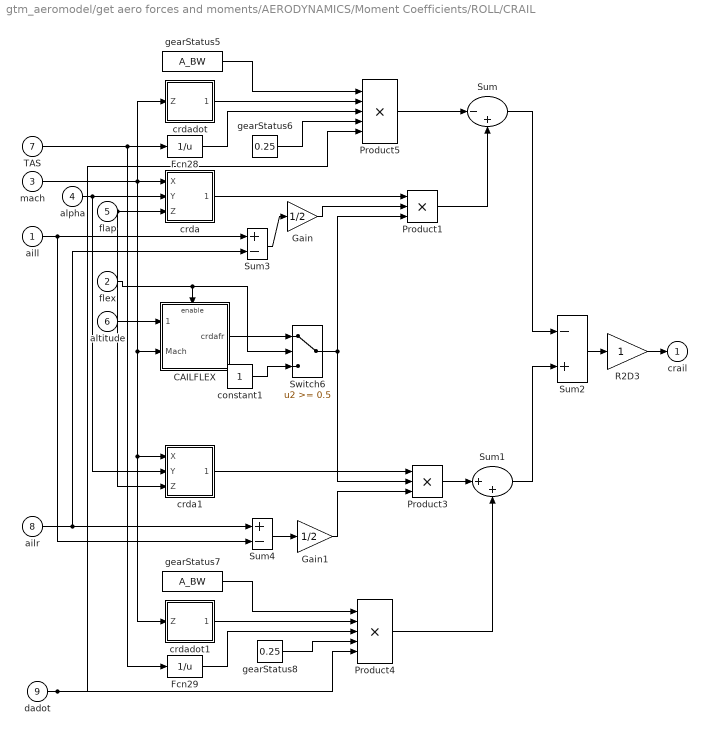
== system gtm_aeromodel/get aero forces and moments/AERODYNAMICS/Moment Coefficients/ROLL/CRAIL ==
  aill : Inport  OutDataType=sfix(16)  OutScaling=2^0
  flex : Inport  Port=2  OutDataType=sfix(16)  OutScaling=2^0
  mach : Inport  Port=3  OutDataType=sfix(16)  OutScaling=2^0
  alpha : Inport  Port=4  OutDataType=sfix(16)  OutScaling=2^0
  flap : Inport  Port=5  OutDataType=sfix(16)  OutScaling=2^0
  altitude : Inport  Port=6  OutDataType=sfix(16)  OutScaling=2^0
  TAS : Inport  Port=7  OutDataType=sfix(16)  OutScaling=2^0
  ailr : Inport  Port=8  OutDataType=sfix(16)  OutScaling=2^0
  dadot : Inport  Port=9  OutDataType=sfix(16)  OutScaling=2^0
  CAILFLEX : Subsystem  TreatAsAtomicUnit=on
  Fcn28 : Fcn  Expr=1/u
  Fcn29 : Fcn  Expr=1/u
  Gain : Gain  Gain=1/2  ParameterDataType=sfix(16)  ParameterScaling=2^0  OutDataType=sfix(16)  OutScaling=2^0  SaturateOnIntegerOverflow=on  OutDataTypeStr=Inherit: Same as input  ParamDataTypeStr=Inherit: Same as input
  Gain1 : Gain  Gain=1/2  ParameterDataType=sfix(16)  ParameterScaling=2^0  OutDataType=sfix(16)  OutScaling=2^0  SaturateOnIntegerOverflow=on  OutDataTypeStr=Inherit: Same as input  ParamDataTypeStr=Inherit: Same as input
  Product1 : Product  Inputs=3  OutDataType=sfix(16)  OutScaling=2^0  SaturateOnIntegerOverflow=on  RndMeth=Zero  InputSameDT=on  OutDataTypeStr=Inherit: Same as first input
  Product3 : Product  Inputs=3  OutDataType=sfix(16)  OutScaling=2^0  SaturateOnIntegerOverflow=on  RndMeth=Zero  InputSameDT=on  OutDataTypeStr=Inherit: Same as first input
  Product4 : Product  Inputs=5  OutDataType=sfix(16)  OutScaling=2^0  SaturateOnIntegerOverflow=on  RndMeth=Zero  InputSameDT=on  OutDataTypeStr=Inherit: Same as first input
  Product5 : Product  Inputs=5  OutDataType=sfix(16)  OutScaling=2^0  SaturateOnIntegerOverflow=on  RndMeth=Zero  InputSameDT=on  OutDataTypeStr=Inherit: Same as first input
  R2D3 : Gain  ParameterDataType=sfix(16)  ParameterScaling=2^0  OutDataType=sfix(16)  OutScaling=2^0  SaturateOnIntegerOverflow=on  OutDataTypeStr=Inherit: Same as input  ParamDataTypeStr=Inherit: Same as input
  Sum : Sum  Inputs=|-+  OutDataType=sfix(16)  OutScaling=2^0  SaturateOnIntegerOverflow=on  InputSameDT=on  OutDataTypeStr=Inherit: Same as first input
  Sum1 : Sum  Inputs=|++  OutDataType=sfix(16)  OutScaling=2^0  SaturateOnIntegerOverflow=on  InputSameDT=on  OutDataTypeStr=Inherit: Same as first input
  Sum2 : Sum  Inputs=-+  OutDataType=sfix(16)  OutScaling=2^0  SaturateOnIntegerOverflow=on  InputSameDT=on  OutDataTypeStr=Inherit: Same as first input
  Sum3 : Sum  Inputs=+-  OutDataType=sfix(16)  OutScaling=2^0  SaturateOnIntegerOverflow=on  InputSameDT=on  OutDataTypeStr=Inherit: Same as first input
  Sum4 : Sum  Inputs=+-  OutDataType=sfix(16)  OutScaling=2^0  SaturateOnIntegerOverflow=on  InputSameDT=on  OutDataTypeStr=Inherit: Same as first input
  Switch6 : Switch  Threshold=0.5  SaturateOnIntegerOverflow=on  InputSameDT=on
  constant1 : Constant  OutDataType=sfix(16)  OutScaling=2^0
  crda : Subsystem  mask(1-2-3 Table){@1=crdax_FMACH, @2=crday_FALPHA, @3=crdaz_FLPDEF, @4=crda}
      mask prompts: @1 "X vector:"; @2 "Y vector:"; @3 "Z vector:"; @4 "Table:"
      mask help: 3-D Table Look Up. Enter monotonic X, Y and Z vectors and a matrix of 2-D tables. See the help for more info.
      mask init:
      | x=@1;y=@2;z=@3;tab=@4;
      mask Help: The X, Y and Z vectors must be monotonic.   The 3-D table is a horizontal concatenation of  2-D tables.  X  indexes into the columns of the 2-D tables & Y indexes into the rows of the 2-D tables.  Z indexes into the table levels (starting with the 1st 2-D table).   The input values are x, y and z respectively (e.g., top port = x).
      mask Display: plot([0 2 2 0 0],[0 0 2 2 0],[0 2 2.9 0.95 0],[2 2 2.7 2.7 2],[2 2.9 2.9 2 2],[0 0.85 2.7 2 0])
  crda1 : Subsystem  mask(1-2-3 Table){@1=crdax_FMACH, @2=crday_FALPHA, @3=crdaz_FLPDEF, @4=crda}
      mask prompts: @1 "X vector:"; @2 "Y vector:"; @3 "Z vector:"; @4 "Table:"
      mask help: 3-D Table Look Up. Enter monotonic X, Y and Z vectors and a matrix of 2-D tables. See the help for more info.
      mask init:
      | x=@1;y=@2;z=@3;tab=@4;
      mask Help: The X, Y and Z vectors must be monotonic.   The 3-D table is a horizontal concatenation of  2-D tables.  X  indexes into the columns of the 2-D tables & Y indexes into the rows of the 2-D tables.  Z indexes into the table levels (starting with the 1st 2-D table).   The input values are x, y and z respectively (e.g., top port = x).
      mask Display: plot([0 2 2 0 0],[0 0 2 2 0],[0 2 2.9 0.95 0],[2 2 2.7 2.7 2],[2 2.9 2.9 2 2],[0 0.85 2.7 2 0])
  crdadot : Subsystem  mask(1-D Table){z=crdadotx_FMACH, tab=crdadot}
      mask prompts: z "Z vector:"; tab "Table:"
      mask help: 1-D Table Look Up. Enter monotonic Z vector amd table. See the help for more info.
      mask Help: The Z vector must be monotonic.  Z indexes into the columns of the 1-D tables.   Table does not extrapolate beyound the break vectors
      mask Display: plot(@2)
  crdadot1 : Subsystem  mask(1-D Table){z=crdadotx_FMACH, tab=crdadot}
      mask prompts: z "Z vector:"; tab "Table:"
      mask help: 1-D Table Look Up. Enter monotonic Z vector amd table. See the help for more info.
      mask Help: The Z vector must be monotonic.  Z indexes into the columns of the 1-D tables.   Table does not extrapolate beyound the break vectors
      mask Display: plot(@2)
  gearStatus5 : Constant  Value=A_BW  OutDataType=sfix(16)  OutScaling=2^0
  gearStatus6 : Constant  Value=0.25  OutDataType=sfix(16)  OutScaling=2^0
  gearStatus7 : Constant  Value=A_BW  OutDataType=sfix(16)  OutScaling=2^0
  gearStatus8 : Constant  Value=0.25  OutDataType=sfix(16)  OutScaling=2^0
  crail : Outport  OutDataType=sfix(16)  OutScaling=2^0  InitialOutput=0
  wires:
  aill/1 -> Sum4/2, Sum3/1
  ailr/1 -> Sum4/1, Sum3/2
  Sum4/1 -> Gain1/1
  Sum3/1 -> Gain/1
  R2D3/1 -> crail/1
  Sum2/1 -> R2D3/1
  gearStatus5/1 -> Product5/1
  crdadot/1(Interp Value) -> Product5/2
  Fcn28/1 -> Product5/3
  gearStatus6/1 -> Product5/4
  dadot/1 -> Product5/5, Product4/5
  Sum1/1 -> Sum2/2
  Sum/1 -> Sum2/1
  Product4/1 -> Sum1/2
  Product3/1 -> Sum1/1
  TAS/1 -> Fcn29/1, Fcn28/1
  Fcn29/1 -> Product4/3
  gearStatus8/1 -> Product4/4
  crdadot1/1(Interp Value) -> Product4/2
  gearStatus7/1 -> Product4/1
  Switch6/1 -> Product3/2, Product1/3
  crda1/1(Interp Value) -> Product3/1
  flap/1 -> crda1/3(Z), crda/3(Z)
  alpha/1 -> crda1/2(Y), crda/2(Y)
  Product1/1 -> Sum/2
  Product5/1 -> Sum/1
  flex/1 -> Switch6/2, CAILFLEX/Enable
  CAILFLEX/1(crdafr) -> Switch6/1
  constant1/1 -> Switch6/3
  altitude/1 -> CAILFLEX/1(altitude)
  mach/1 -> crdadot1/1(Z), crda1/1(X), CAILFLEX/2(Mach), crdadot/1(Z), crda/1(X)
  crda/1(Interp Value) -> Product1/1
  Gain/1 -> Product1/2
  Gain1/1 -> Product3/3

== system gtm_aeromodel/get aero forces and moments/AERODYNAMICS/Moment Coefficients/ROLL/CRBWB ==
  alpha : Inport  OutDataType=sfix(16)  OutScaling=2^0
  mach : Inport  Port=2  OutDataType=sfix(16)  OutScaling=2^0
  flap : Inport  Port=3  OutDataType=sfix(16)  OutScaling=2^0
  flex : Inport  Port=4  OutDataType=sfix(16)  OutScaling=2^0
  altitude : Inport  Port=5  OutDataType=sfix(16)  OutScaling=2^0
  CRWBFLEX : Subsystem  TreatAsAtomicUnit=on
  Sum : Sum  OutDataType=sfix(16)  OutScaling=2^0  SaturateOnIntegerOverflow=on  InputSameDT=on  OutDataTypeStr=Inherit: Same as first input
  Switch5 : Switch  Threshold=0.1  SaturateOnIntegerOverflow=on  InputSameDT=on
  constant : Constant  Value=0.0  OutDataType=sfix(16)  OutScaling=2^0
  cr_flap_ : Subsystem  TreatAsAtomicUnit=on
  crbwb_ : Subsystem  mask(2-D Table){y=crbwbx_FMACH, z=crbwby_FALPHA, tab=crbwb}
      mask prompts: y "Y vector:"; z "Z vector:"; tab "Table:"
      mask help: 2-D Table Look Up. Enter monotonic Y and Z vectors and a matrix of 2-D tables. See the help for more info.
      mask Help: The Y and Z vectors must be monotonic.  Y  indexes into the columns of the 2-D table & Z indexes into the rows of the 2-D tables.   The input values are y and z respectively (e.g., top port = y).
      mask Display: plot(-10,-10,110,110,[90,50,10],[90,40,30],[90,50,10],[50,26,20],[90,50,10],[22,13,10])
  crbwb_fl : Outport  OutDataType=sfix(16)  OutScaling=2^0  InitialOutput=0
  crbfr : Outport  Port=2  OutDataType=sfix(16)  OutScaling=2^0  InitialOutput=0
  wires:
  crbwb_/1(Interp Value) -> Sum/2
  CRWBFLEX/1(crbfr) -> crbfr/1
  flex/1 -> CRWBFLEX/Enable
  Switch5/1 -> Sum/1
  constant/1 -> Switch5/3
  mach/1 -> CRWBFLEX/2(Mach), crbwb_/1(Y)
  altitude/1 -> CRWBFLEX/1(altitude)
  cr_flap_/1(cr_flap) -> Switch5/1
  flap/1 -> cr_flap_/1(flap), Switch5/2, cr_flap_/Enable
  Sum/1 -> crbwb_fl/1
  alpha/1 -> cr_flap_/2(alpha), crbwb_/2(Z)

== system gtm_aeromodel/get aero forces and moments/AERODYNAMICS/Moment Coefficients/ROLL/CRGEAR ==
  flap : Inport  OutDataType=sfix(16)  OutScaling=2^0
  gear : Inport  Port=2  OutDataType=sfix(16)  OutScaling=2^0
  beta : Inport  Port=3  OutDataType=sfix(16)  OutScaling=2^0
  Product1 : Product  OutDataType=sfix(16)  OutScaling=2^0  SaturateOnIntegerOverflow=on  RndMeth=Zero  InputSameDT=on  OutDataTypeStr=Inherit: Same as first input
  Switch6 : Switch  Threshold=0.5  SaturateOnIntegerOverflow=on  InputSameDT=on
  constant1 : Constant  Value=0.0  OutDataType=sfix(16)  OutScaling=2^0
  dcrb_ : Subsystem  mask(1-D Table){z=dcrbx_FLPDEF, tab=dcrb}
      mask prompts: z "Z vector:"; tab "Table:"
      mask help: 1-D Table Look Up. Enter monotonic Z vector amd table. See the help for more info.
      mask Help: The Z vector must be monotonic.  Z indexes into the columns of the 1-D tables.   Table does not extrapolate beyound the break vectors
      mask Display: plot(@2)
  crg : Outport  OutDataType=sfix(16)  OutScaling=2^0  InitialOutput=0
  wires:
  dcrb_/1(Interp Value) -> Product1/2
  flap/1 -> dcrb_/1(Z)
  gear/1 -> Switch6/2
  constant1/1 -> Switch6/3
  Switch6/1 -> crg/1
  beta/1 -> Product1/1
  Product1/1 -> Switch6/1

== system gtm_aeromodel/get aero forces and moments/AERODYNAMICS/Moment Coefficients/ROLL/CRP ==
  mach : Inport  OutDataType=sfix(16)  OutScaling=2^0
  alpha : Inport  Port=2  OutDataType=sfix(16)  OutScaling=2^0
  altitude : Inport  Port=3  OutDataType=sfix(16)  OutScaling=2^0
  flex : Inport  Port=4  OutDataType=sfix(16)  OutScaling=2^0
  phat : Inport  Port=5  OutDataType=sfix(16)  OutScaling=2^0
  CRPFLEX : Subsystem  TreatAsAtomicUnit=on
  Fcn28 : Fcn  Expr=1/u
  Product3 : Product  OutDataType=sfix(16)  OutScaling=2^0  SaturateOnIntegerOverflow=on  RndMeth=Zero  InputSameDT=on  OutDataTypeStr=Inherit: Same as first input
  Switch7 : Switch  Threshold=0.5  SaturateOnIntegerOverflow=on  InputSameDT=on
  constant : Constant  OutDataType=sfix(16)  OutScaling=2^0
  constant2 : Constant  Value=2  OutDataType=sfix(16)  OutScaling=2^0
  constant3 : Constant  Value=constants.r2d  OutDataType=sfix(16)  OutScaling=2^0
  crp : Product  Inputs=4  OutDataType=sfix(16)  OutScaling=2^0  SaturateOnIntegerOverflow=on  RndMeth=Zero  InputSameDT=on  OutDataTypeStr=Inherit: Same as first input
  crptail : Product  OutDataType=sfix(16)  OutScaling=2^0  SaturateOnIntegerOverflow=on  RndMeth=Zero  InputSameDT=on  OutDataTypeStr=Inherit: Same as first input
  crptot : Sum  Inputs=|++  OutDataType=sfix(16)  OutScaling=2^0  SaturateOnIntegerOverflow=on  InputSameDT=on  OutDataTypeStr=Inherit: Same as first input
  crpwb : Product  OutDataType=sfix(16)  OutScaling=2^0  SaturateOnIntegerOverflow=on  RndMeth=Zero  InputSameDT=on  OutDataTypeStr=Inherit: Same as first input
  crpwb_ : Subsystem  mask(2-D Table){y=crpwbx_FMACH, z=crpwby_FALPHA, tab=crpwb}
      mask prompts: y "Y vector:"; z "Z vector:"; tab "Table:"
      mask help: 2-D Table Look Up. Enter monotonic Y and Z vectors and a matrix of 2-D tables. See the help for more info.
      mask Help: The Y and Z vectors must be monotonic.  Y  indexes into the columns of the 2-D table & Z indexes into the rows of the 2-D tables.   The input values are y and z respectively (e.g., top port = y).
      mask Display: plot(-10,-10,110,110,[90,50,10],[90,40,30],[90,50,10],[50,26,20],[90,50,10],[22,13,10])
  dcyrt : Product  OutDataType=sfix(16)  OutScaling=2^0  SaturateOnIntegerOverflow=on  RndMeth=Zero  InputSameDT=on  OutDataTypeStr=Inherit: Same as first input
  rcrbvt : Subsystem  mask(2-D Table){y=crbvtx_FMACH, z=crbvty_FALPHA, tab=crbvt}
      mask prompts: y "Y vector:"; z "Z vector:"; tab "Table:"
      mask help: 2-D Table Look Up. Enter monotonic Y and Z vectors and a matrix of 2-D tables. See the help for more info.
      mask Help: The Y and Z vectors must be monotonic.  Y  indexes into the columns of the 2-D table & Z indexes into the rows of the 2-D tables.   The input values are y and z respectively (e.g., top port = y).
      mask Display: plot(-10,-10,110,110,[90,50,10],[90,40,30],[90,50,10],[50,26,20],[90,50,10],[22,13,10])
  rcybvt : Subsystem  mask(2-D Table){y=cybvtx_FMACH, z=cybvty_FALPHA, tab=cybvt}
      mask prompts: y "Y vector:"; z "Z vector:"; tab "Table:"
      mask help: 2-D Table Look Up. Enter monotonic Y and Z vectors and a matrix of 2-D tables. See the help for more info.
      mask Help: The Y and Z vectors must be monotonic.  Y  indexes into the columns of the 2-D table & Z indexes into the rows of the 2-D tables.   The input values are y and z respectively (e.g., top port = y).
      mask Display: plot(-10,-10,110,110,[90,50,10],[90,40,30],[90,50,10],[50,26,20],[90,50,10],[22,13,10])
  dcrphat : Outport  OutDataType=sfix(16)  OutScaling=2^0  InitialOutput=0
  wires:
  constant3/1 -> crp/1
  crpwb/1 -> crptot/2
  crpwb_/1(Interp Value) -> crpwb/1
  Switch7/1 -> crpwb/2, crptail/2
  crptot/1 -> dcyrt/1
  phat/1 -> dcyrt/2
  dcyrt/1 -> dcrphat/1
  crptail/1 -> crptot/1
  crp/1 -> crptail/1
  Product3/1 -> crp/2
  rcrbvt/1(Interp Value) -> Product3/2, Product3/1
  Fcn28/1 -> crp/3
  alpha/1 -> crpwb_/2(Z), rcrbvt/2(Z), rcybvt/2(Z)
  altitude/1 -> CRPFLEX/1(altitude)
  flex/1 -> CRPFLEX/Enable, Switch7/2
  mach/1 -> rcrbvt/1(Y), rcybvt/1(Y), CRPFLEX/2(Mach), crpwb_/1(Y)
  constant2/1 -> crp/4
  CRPFLEX/1(crpfr) -> Switch7/1
  constant/1 -> Switch7/3
  rcybvt/1(Interp Value) -> Fcn28/1
